simulink model "HeatExchanger"  (Simulink 7.7)
settings: Solver=ode45  StartTime=0.0  StopTime=500  RelTol=1e-3
InitFcn:
  | HeatExchangerParameters
StartFcn:
  | HeatExchangerParameters
values from neighbouring files (symbols this model uses):
  A = 1    [HeatExchangerParameters.m]
  k = 0.1    [HeatExchangerParameters.m]
  m = 100    [HeatExchangerParameters.m]
  N = 10    [HeatExchangerParameters.m]
  T_init = 300    [HeatExchangerParameters.m]
settings Model: Creator=simon  LastModifiedBy=simon

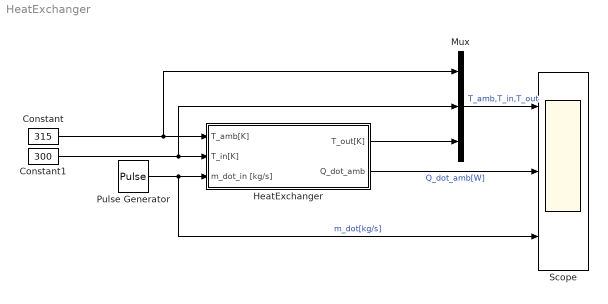
== system HeatExchanger ==
  Constant : Constant  Value=315
  Constant1 : Constant  Value=300
  HeatExchanger : Subsystem
  Mux : Mux  Inputs=3
  Pulse Generator : DiscretePulseGenerator  PulseType=Time based  Period=60  PulseWidth=40
  Scope : Scope  NumInputPorts=3
      settings: TickLabels=on  YMin=-5~-5~-5  YMax=5~5~5
  wires:
  Mux/1 -> Scope/1  "T_amb,T_in,T_out"
  HeatExchanger/1(T_out[K]) -> Mux/3
  HeatExchanger/2(Q_dot_amb) -> Scope/2  "Q_dot_amb[W]"
  Constant/1 -> HeatExchanger/1(T_amb[K]), Mux/1
  Pulse Generator/1 -> HeatExchanger/3(m_dot_in [kg/s]), Scope/3  "m_dot[kg/s]"
  Constant1/1 -> HeatExchanger/2(T_in[K]), Mux/2

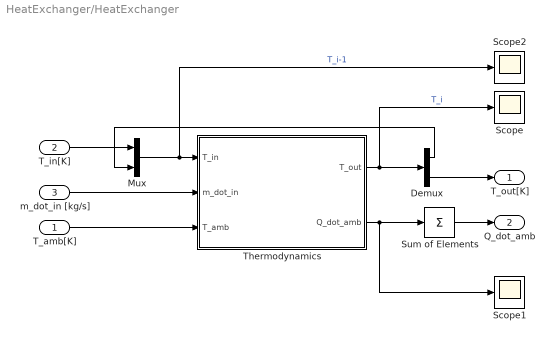
== system HeatExchanger/HeatExchanger ==
  T_amb[K] : Inport
  T_in[K] : Inport  Port=2
  m_dot_in [kg/s] : Inport  Port=3
  Demux : Demux  Outputs=[-1 1]
  Mux : Mux  Inputs=[1 -1]
  Scope : Scope
  Scope1 : Scope
      settings: SaveName=ScopeData2
  Scope2 : Scope
      settings: SaveName=ScopeData3
  Sum of Elements : Sum  Inputs=+
  Thermodynamics : Subsystem
  T_out[K] : Outport
  Q_dot_amb : Outport  Port=2
  wires:
  T_in[K]/1 -> Mux/1
  Demux/2 -> T_out[K]/1
  m_dot_in [kg/s]/1 -> Thermodynamics/2(m_dot_in)
  Mux/1 -> Thermodynamics/1(T_in), Scope2/1  "T_i-1"
  Sum of Elements/1 -> Q_dot_amb/1
  T_amb[K]/1 -> Thermodynamics/3(T_amb)
  Thermodynamics/1(T_out) -> Demux/1, Scope/1  "T_i"
  Thermodynamics/2(Q_dot_amb) -> Sum of Elements/1, Scope1/1
  Demux/1 -> Mux/2

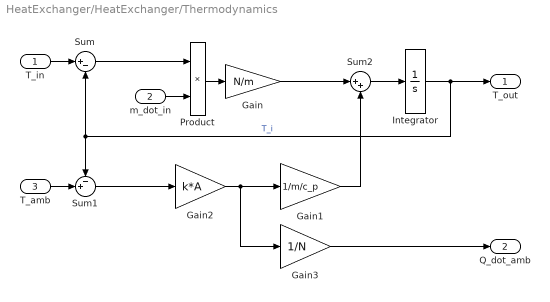
== system HeatExchanger/HeatExchanger/Thermodynamics ==
  T_in : Inport
  m_dot_in : Inport  Port=2
  T_amb : Inport  Port=3
  Gain : Gain  Gain=N/m
  Gain1 : Gain  Gain=1/m/c_p
  Gain2 : Gain  Gain=k*A
  Gain3 : Gain  Gain=1/N
  Integrator : Integrator  InitialCondition=T_init*ones(N,1)  ContinuousStateAttributes='T'
  Product : Product  RndMeth=Zero
  Sum : Sum  Inputs=|+-
  Sum1 : Sum  Inputs=-+|
  Sum2 : Sum  Inputs=|++
  T_out : Outport
  Q_dot_amb : Outport  Port=2
  wires:
  Integrator/1 -> Sum/2, Sum1/1, T_out/1  "T_i"
  Product/1 -> Gain/1
  Sum/1 -> Product/1
  Sum1/1 -> Gain2/1
  Gain1/1 -> Sum2/2
  Sum2/1 -> Integrator/1
  Gain/1 -> Sum2/1
  T_in/1 -> Sum/1
  m_dot_in/1 -> Product/2
  T_amb/1 -> Sum1/2
  Gain2/1 -> Gain1/1, Gain3/1
  Gain3/1 -> Q_dot_amb/1
